simulink model "ASSIG2_vFinal"  (R2020a)
settings: Solver=FixedStepAuto  StartTime=0.0  StopTime=10.0  FixedStep=1e-3  RelTol=1e-3  EnableMultiTasking=on
undefined symbols (not defined in the file): A0, A1, D0, D1, D10, D11, D12, D13, D2, D3, D4, D5, D6, D7, D8, D9, PTA0, PTA1, PTA2, PTB2, PTB23, PTB3, PTB9, PTC16, PTC17, PTC2, PTC3, PTC4, PTD0, PTD1, PTD2, PTD3
libraries: etargetslib x22, frdmk64flib x19
settings Model: ExtModeTrigDuration=5  Creator=Nour  LastModifiedBy=Daniyal
settings OptimizationCC: EnhancedBackFolding=on  PassReuseOutputArgsAs=Individual arguments  ZeroExternalMemoryAtStartup=off  ZeroInternalMemoryAtStartup=off  MaxStackSize=64  OptimizeBlockOrder=speed  DifferentSizesBufferReuse=on  OptimizationCustomize=off  EfficientTunableParamExpr=on
settings DebuggingCC: ParameterTunabilityLossMsg=error
settings HardwareCC: ProdBitPerPointer=32  ProdBitPerSizeT=32  ProdBitPerPtrDiffT=32  ProdLargestAtomicInteger=Long  ProdLargestAtomicFloat=Double  ProdWordSize=32  ProdHWDeviceType=ARM Compatible->ARM Cortex
settings SFSimCC: MATLABDynamicMemAlloc=off
settings RTWCC: SystemTargetFile=ert.tlc  HardwareBoard=NXP FRDM-K64F  TemplateMakefile=ert_default_tmf  Toolchain=GNU Tools for ARM Embedded Processors
settings CodeAppCC: ForceParamTrailComments=on  IgnoreCustomStorageClasses=off  OperatorAnnotations=on  SimulinkDataObjDesc=on  SFDataObjDesc=on  InsertBlockDesc=on

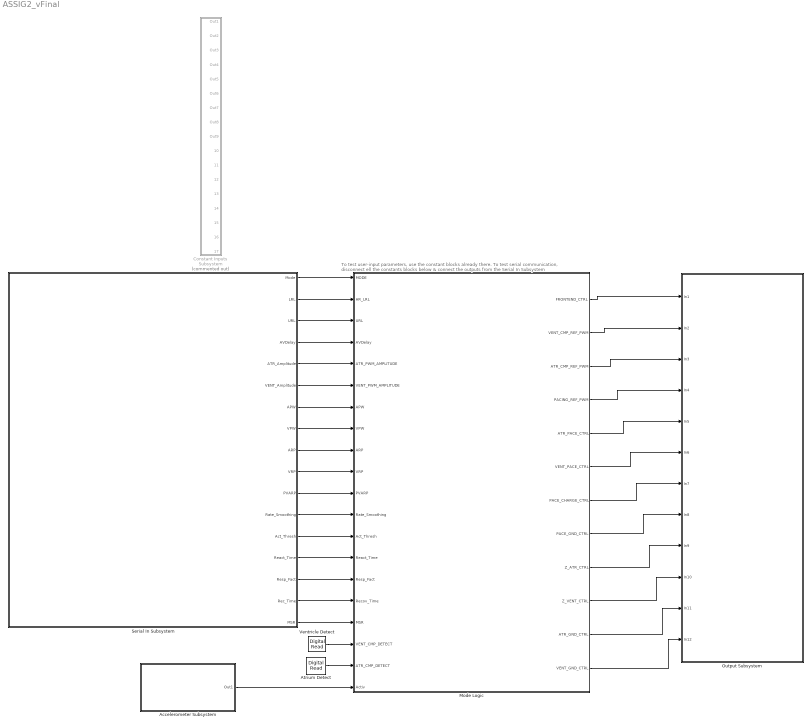
== system ASSIG2_vFinal ==
  note: To test user-input parameters, use the constant blocks already there.
      | To test serial communication, disconnect ell the constants blocks below & connect the outputs from the Serial In Subsystem
  Accelerometer Subsystem : Subsystem
  Atrium Detect : frdmk64flib/Digital Read  Whichpin=PTC16 (D0)  SampleTime=-1
  Constant Inputs Subsystem : Subsystem  Commented=on
  Mode Logic : Stateflow chart  TreatAsAtomicUnit=on
  Output Subsystem : Subsystem
  Serial In Subsystem : Subsystem
  Ventricle Detect : frdmk64flib/Digital Read  Whichpin=PTC17 (D1)  SampleTime=-1
  wires:
  Ventricle Detect/1 -> Mode Logic/18(VENT_CMP_DETECT)
  Atrium Detect/1 -> Mode Logic/19(ATR_CMP_DETECT)
  Mode Logic/1(FRONTEND_CTRL) -> Output Subsystem/1(In1)
  Mode Logic/2(VENT_CMP_REF_PWM) -> Output Subsystem/2(In2)
  Mode Logic/3(ATR_CMP_REF_PWM) -> Output Subsystem/3(In3)
  Mode Logic/4(PACING_REF_PWM) -> Output Subsystem/4(In4)
  Mode Logic/5(ATR_PACE_CTRL) -> Output Subsystem/5(In5)
  Mode Logic/6(VENT_PACE_CTRL) -> Output Subsystem/6(In6)
  Mode Logic/7(PACE_CHARGE_CTRL) -> Output Subsystem/7(In7)
  Mode Logic/8(PACE_GND_CTRL) -> Output Subsystem/8(In8)
  Mode Logic/9(Z_ATR_CTRL) -> Output Subsystem/9(In9)
  Mode Logic/10(Z_VENT_CTRL) -> Output Subsystem/10(In10)
  Mode Logic/11(ATR_GND_CTRL) -> Output Subsystem/11(In11)
  Mode Logic/12(VENT_GND_CTRL) -> Output Subsystem/12(In12)
  Serial In Subsystem/3(URL) -> Mode Logic/3(URL)
  Serial In Subsystem/4(AVDelay) -> Mode Logic/4(AVDelay)
  Serial In Subsystem/5(ATR_Amplitude) -> Mode Logic/5(ATR_PWM_AMPLITUDE)
  Serial In Subsystem/6(VENT_Amplitude) -> Mode Logic/6(VENT_PWM_AMPLITUDE)
  Serial In Subsystem/7(APW) -> Mode Logic/7(APW)
  Serial In Subsystem/8(VPW) -> Mode Logic/8(VPW)
  Serial In Subsystem/9(ARP) -> Mode Logic/9(ARP)
  Serial In Subsystem/10(VRP) -> Mode Logic/10(VRP)
  Serial In Subsystem/11(PVARP) -> Mode Logic/11(PVARP)
  Serial In Subsystem/12(Rate_Smoothing) -> Mode Logic/12(Rate_Smoothing)
  Serial In Subsystem/13(Act_Thresh) -> Mode Logic/13(Act_Thresh)
  Serial In Subsystem/14(React_Time) -> Mode Logic/14(React_Time)
  Serial In Subsystem/15(Resp_Fact) -> Mode Logic/15(Resp_Fact)
  Serial In Subsystem/16(Rec_Time) -> Mode Logic/16(Recov_Time)
  Serial In Subsystem/17(MSR) -> Mode Logic/17(MSR)
  Accelerometer Subsystem/1(Out1) -> Mode Logic/20(Activ)
  Serial In Subsystem/2(LRL) -> Mode Logic/2(HR_LRL)
  Serial In Subsystem/1(Mode) -> Mode Logic/1(MODE)

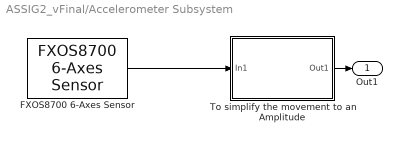
== system ASSIG2_vFinal/Accelerometer Subsystem ==
  FXOS8700 6-Axes Sensor : frdmk64flib/FXOS8700 6-Axes Sensor  Activesensor=Accelerometer only  ODR=800Hz  HybridODR=400Hz  Accelfullrange=-4g to +4g  SampleTime=-1
  To simplify the movement to an Amplitude : Subsystem
  Out1 : Outport
  wires:
  FXOS8700 6-Axes Sensor/1 -> To simplify the movement to an Amplitude/1(In1)
  To simplify the movement to an Amplitude/1(Out1) -> Out1/1

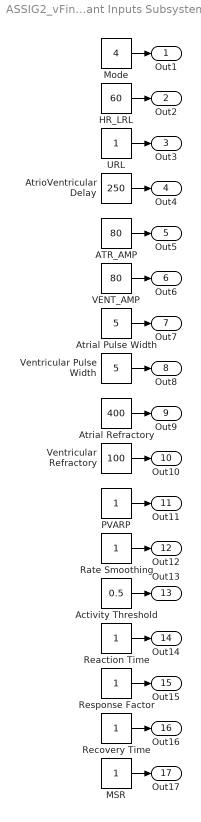
== system ASSIG2_vFinal/Constant Inputs Subsystem ==
  ATR_AMP : Constant  Value=80  OutDataTypeStr=uint8
  Activity Threshold : Constant  Value=0.5  OutDataTypeStr=single
  Atrial Pulse Width : Constant  Value=5  OutDataTypeStr=uint16
  Atrial Refractory : Constant  Value=400  OutDataTypeStr=uint16
  AtrioVentricular Delay : Constant  Value=250  OutDataTypeStr=uint16
  HR_LRL : Constant  Value=60  OutDataTypeStr=uint16
  MSR : Constant  OutDataTypeStr=uint16
  Mode : Constant  Value=4  OutDataTypeStr=uint8
  PVARP : Constant  OutDataTypeStr=uint16
  Rate Smoothing : Constant  OutDataTypeStr=uint8
  Reaction Time : Constant  OutDataTypeStr=uint16
  Recovery Time : Constant  OutDataTypeStr=uint16
  Response Factor : Constant  OutDataTypeStr=uint16
  URL : Constant  OutDataTypeStr=uint8
  VENT_AMP : Constant  Value=80  OutDataTypeStr=uint8
  Ventricular Pulse Width : Constant  Value=5  OutDataTypeStr=uint16
  Ventricular Refractory : Constant  Value=100  OutDataTypeStr=uint16
  Out1 : Outport
  Out2 : Outport  Port=2
  Out3 : Outport  Port=3
  Out4 : Outport  Port=4
  Out5 : Outport  Port=5
  Out6 : Outport  Port=6
  Out7 : Outport  Port=7
  Out8 : Outport  Port=8
  Out9 : Outport  Port=9
  Out10 : Outport  Port=10
  Out11 : Outport  Port=11
  Out12 : Outport  Port=12
  Out13 : Outport  Port=13
  Out14 : Outport  Port=14
  Out15 : Outport  Port=15
  Out16 : Outport  Port=16
  Out17 : Outport  Port=17
  wires:
  VENT_AMP/1 -> Out6/1
  Response Factor/1 -> Out15/1
  URL/1 -> Out3/1
  Recovery Time/1 -> Out16/1
  Ventricular Refractory/1 -> Out10/1
  Atrial Pulse Width/1 -> Out7/1
  Rate Smoothing/1 -> Out12/1
  Atrial Refractory/1 -> Out9/1
  Activity Threshold/1 -> Out13/1
  AtrioVentricular Delay/1 -> Out4/1
  Mode/1 -> Out1/1
  Ventricular Pulse Width/1 -> Out8/1
  Reaction Time/1 -> Out14/1
  HR_LRL/1 -> Out2/1
  PVARP/1 -> Out11/1
  MSR/1 -> Out17/1
  ATR_AMP/1 -> Out5/1

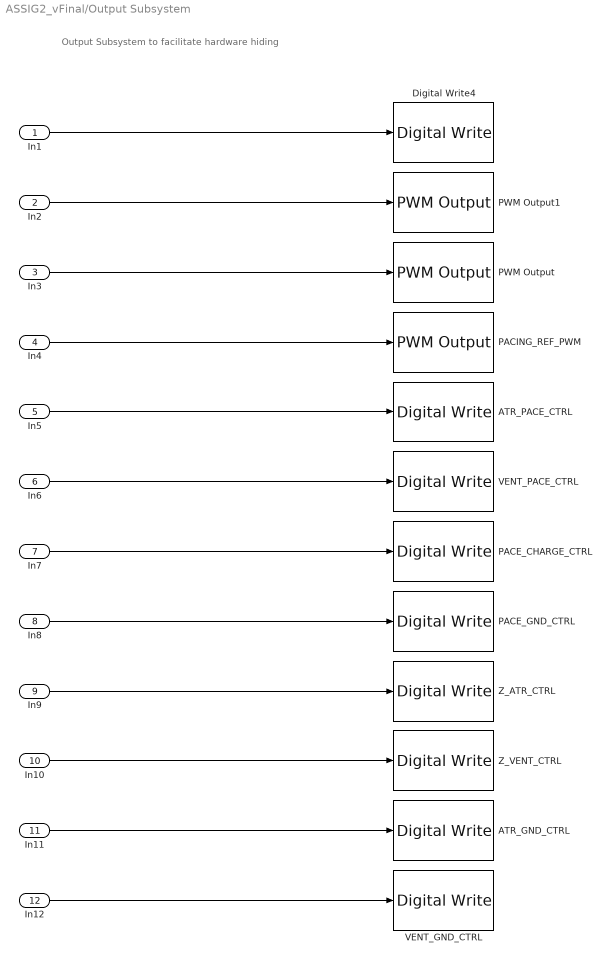
== system ASSIG2_vFinal/Output Subsystem ==
  note: Output Subsystem to facilitate hardware hiding
  In1 : Inport
  In2 : Inport  Port=2
  In3 : Inport  Port=3
  In4 : Inport  Port=4
  In5 : Inport  Port=5
  In6 : Inport  Port=6
  In7 : Inport  Port=7
  In8 : Inport  Port=8
  In9 : Inport  Port=9
  In10 : Inport  Port=10
  In11 : Inport  Port=11
  In12 : Inport  Port=12
  ATR_GND_CTRL : frdmk64flib/Digital Write  Whichpin=PTD2 (D11)
  ATR_PACE_CTRL : frdmk64flib/Digital Write  Whichpin=PTA0 (D8)
  Digital Write4 : frdmk64flib/Digital Write  Whichpin=PTD1 (D13)
  PACE_CHARGE_CTRL : frdmk64flib/Digital Write  Whichpin=PTB9 (D2)
  PACE_GND_CTRL : frdmk64flib/Digital Write  Whichpin=PTD0 (D10)
  PACING_REF_PWM : frdmk64flib/PWM Output  Whichpin=PTA2 (D5)  InitialFrequency=2000  InitialDutyCycle=80
  PWM Output : frdmk64flib/PWM Output  Whichpin=PTC2 (D6)  InitialFrequency=2000  InitialDutyCycle=20
  PWM Output1 : frdmk64flib/PWM Output  Whichpin=PTA1 (D3)  InitialFrequency=2000  InitialDutyCycle=40
  VENT_GND_CTRL : frdmk64flib/Digital Write  Whichpin=PTD3 (D12)
  VENT_PACE_CTRL : frdmk64flib/Digital Write  Whichpin=PTC4 (D9)
  Z_ATR_CTRL : frdmk64flib/Digital Write  Whichpin=PTB23 (D4)
  Z_VENT_CTRL : frdmk64flib/Digital Write  Whichpin=PTC3 (D7)
  wires:
  In7/1 -> PACE_CHARGE_CTRL/1
  In12/1 -> VENT_GND_CTRL/1
  In1/1 -> Digital Write4/1
  In4/1 -> PACING_REF_PWM/1
  In8/1 -> PACE_GND_CTRL/1
  In6/1 -> VENT_PACE_CTRL/1
  In9/1 -> Z_ATR_CTRL/1
  In10/1 -> Z_VENT_CTRL/1
  In11/1 -> ATR_GND_CTRL/1
  In2/1 -> PWM Output1/1
  In5/1 -> ATR_PACE_CTRL/1
  In3/1 -> PWM Output/1

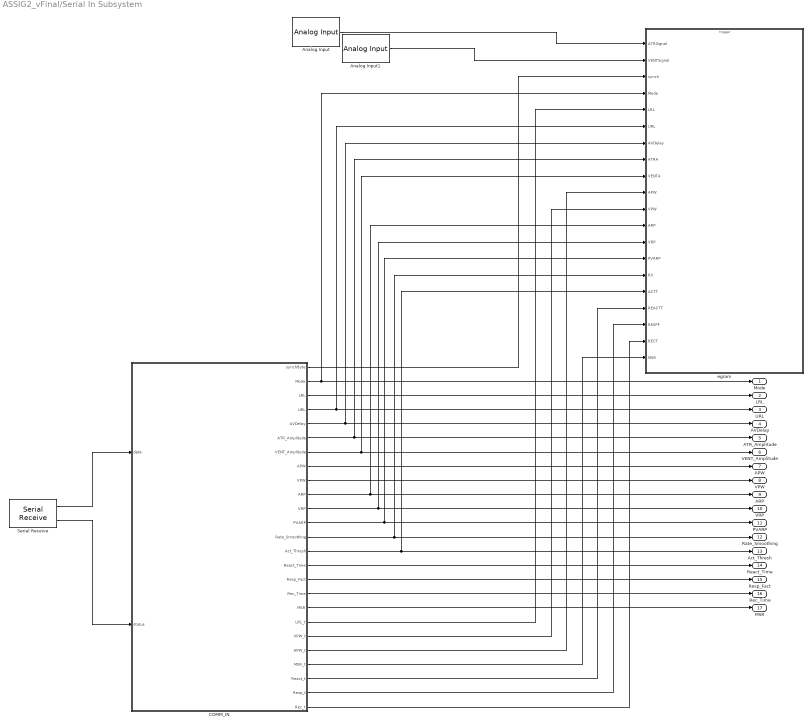
== system ASSIG2_vFinal/Serial In Subsystem ==
  Analog Input : frdmk64flib/Analog Input  Whichpin=PTB2 (A0)  SampleTime=-1
  Analog Input1 : frdmk64flib/Analog Input  Whichpin=PTB3 (A1)  SampleTime=-1
  COMM_IN : Stateflow chart  TreatAsAtomicUnit=on
  Serial Receive : frdmk64flib/Serial Receive  SCIModule=0  Baudrate=uint32(9600)  Parity=None  StopBits=1  HardwareFlowControl=None  ByteOrder=LittleEndian  DataType=uint8  DataLength=26  BlockingMode=off  OutputStatus=on  SampleTime=-1
  egram : Subsystem
  Mode : Outport
  LRL : Outport  Port=2
  URL : Outport  Port=3
  AVDelay : Outport  Port=4
  ATR_Amplitude : Outport  Port=5
  VENT_Amplitude : Outport  Port=6
  APW : Outport  Port=7
  VPW : Outport  Port=8
  ARP : Outport  Port=9
  VRP : Outport  Port=10
  PVARP : Outport  Port=11
  Rate_Smoothing : Outport  Port=12
  Act_Thresh : Outport  Port=13
  React_Time : Outport  Port=14
  Resp_Fact : Outport  Port=15
  Rec_Time : Outport  Port=16
  MSR : Outport  Port=17
  wires:
  Serial Receive/1 -> COMM_IN/1(data)
  Serial Receive/2 -> COMM_IN/2(status)
  Analog Input/1 -> egram/1(ATRSignal)
  Analog Input1/1 -> egram/2(VENTSignal)
  COMM_IN/2(Mode) -> Mode/1, egram/4(Mode)
  COMM_IN/3(LRL) -> LRL/1
  COMM_IN/4(URL) -> URL/1, egram/6(URL)
  COMM_IN/5(AVDelay) -> AVDelay/1, egram/7(AVDelay)
  COMM_IN/6(ATR_Amplitude) -> egram/8(ATRA), ATR_Amplitude/1
  COMM_IN/7(VENT_Amplitude) -> egram/9(VENTA), VENT_Amplitude/1
  COMM_IN/8(APW) -> APW/1
  COMM_IN/9(VPW) -> VPW/1
  COMM_IN/10(ARP) -> egram/12(ARP), ARP/1
  COMM_IN/18(MSR) -> MSR/1
  COMM_IN/17(Rec_Time) -> Rec_Time/1
  COMM_IN/16(Resp_Fact) -> Resp_Fact/1
  COMM_IN/15(React_Time) -> React_Time/1
  COMM_IN/14(Act_Thresh) -> egram/16(ACTT), Act_Thresh/1
  COMM_IN/13(Rate_Smoothing) -> egram/15(RS), Rate_Smoothing/1
  COMM_IN/12(PVARP) -> egram/14(PVARP), PVARP/1
  COMM_IN/11(VRP) -> egram/13(VRP), VRP/1
  COMM_IN/1(synchByte) -> egram/3(synch)
  COMM_IN/19(LRL_t) -> egram/5(LRL)
  COMM_IN/20(VPW_t) -> egram/11(VPW)
  COMM_IN/21(APW_t) -> egram/10(APW)
  COMM_IN/23(React_t) -> egram/17(REACTT)
  COMM_IN/24(Resp_t) -> egram/18(RESPF)
  COMM_IN/25(Rec_t) -> egram/19(RECT)
  COMM_IN/22(MSR_t) -> egram/20(MSR)

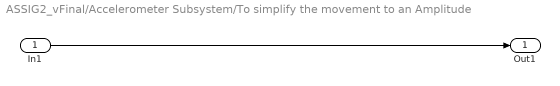
== system ASSIG2_vFinal/Accelerometer Subsystem/To simplify the movement to an Amplitude ==
  In1 : Inport
  Out1 : Outport
  wires:
  In1/1 -> Out1/1

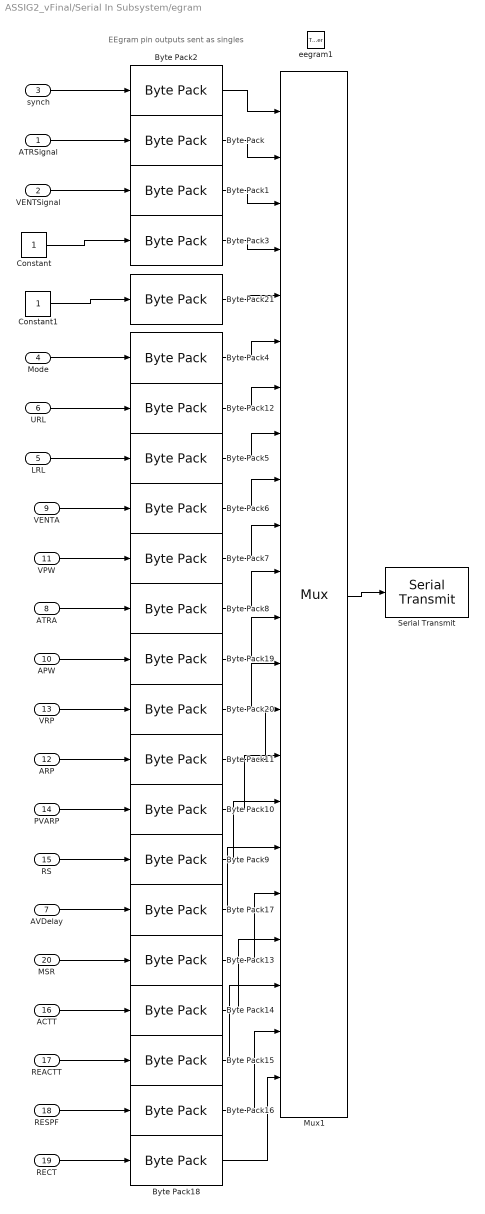
== system ASSIG2_vFinal/Serial In Subsystem/egram ==
  note: EEgram pin outputs sent as singles
  ATRSignal : Inport
  VENTSignal : Inport  Port=2
  synch : Inport  Port=3
  Mode : Inport  Port=4
  LRL : Inport  Port=5
  URL : Inport  Port=6
  AVDelay : Inport  Port=7
  ATRA : Inport  Port=8
  VENTA : Inport  Port=9
  APW : Inport  Port=10
  VPW : Inport  Port=11
  ARP : Inport  Port=12
  VRP : Inport  Port=13
  PVARP : Inport  Port=14
  RS : Inport  Port=15
  ACTT : Inport  Port=16
  REACTT : Inport  Port=17
  RESPF : Inport  Port=18
  RECT : Inport  Port=19
  MSR : Inport  Port=20
  eegram1 : TriggerPort  TriggerType=function-call  IsSimulinkFunction=on  FunctionName=eegram1  VariantControl=Variant  PortDimensions=1
  Byte Pack : etargetslib/Byte Pack  datatypes={'double'}  byteAlign=1
  Byte Pack1 : etargetslib/Byte Pack  datatypes={'double'}  byteAlign=1
  Byte Pack{3,10..11,17,20} (5 alike) : etargetslib/Byte Pack  datatypes={'uint16'}  byteAlign=1
  Byte Pack{2,4..9,12..13,15..16,18..19} (13 alike) : etargetslib/Byte Pack  datatypes={'uint8'}  byteAlign=1
  Byte Pack14 : etargetslib/Byte Pack  datatypes={'single'}  byteAlign=1
  Byte Pack21 : etargetslib/Byte Pack  datatypes={'single'}  byteAlign=1
  Constant : Constant  OutDataTypeStr=uint16
  Constant1 : Constant  OutDataTypeStr=single
  Mux1 : Mux  Inputs=22
  Serial Transmit : frdmk64flib/Serial Transmit  SCIModule=0  Baudrate=uint32(9600)  Parity=None  StopBits=1  HardwareFlowControl=None  ByteOrder=LittleEndian  BlockingMode=on  OutputStatus=off
  wires:
  ATRSignal/1 -> Byte Pack/1
  VENTSignal/1 -> Byte Pack1/1
  Mode/1 -> Byte Pack4/1
  ARP/1 -> Byte Pack11/1
  synch/1 -> Byte Pack2/1
  ACTT/1 -> Byte Pack14/1
  PVARP/1 -> Byte Pack10/1
  VENTA/1 -> Byte Pack6/1
  MSR/1 -> Byte Pack13/1
  AVDelay/1 -> Byte Pack17/1
  REACTT/1 -> Byte Pack15/1
  LRL/1 -> Byte Pack5/1
  VRP/1 -> Byte Pack20/1
  ATRA/1 -> Byte Pack8/1
  APW/1 -> Byte Pack19/1
  RS/1 -> Byte Pack9/1
  VPW/1 -> Byte Pack7/1
  URL/1 -> Byte Pack12/1
  RESPF/1 -> Byte Pack16/1
  RECT/1 -> Byte Pack18/1
  Byte Pack2/1 -> Mux1/1
  Byte Pack/1 -> Mux1/2
  Byte Pack1/1 -> Mux1/3
  Mux1/1 -> Serial Transmit/1
  Constant/1 -> Byte Pack3/1
  Byte Pack3/1 -> Mux1/4
  Byte Pack21/1 -> Mux1/5
  Byte Pack4/1 -> Mux1/6
  Byte Pack12/1 -> Mux1/7
  Byte Pack5/1 -> Mux1/8
  Byte Pack6/1 -> Mux1/9
  Byte Pack7/1 -> Mux1/10
  Byte Pack8/1 -> Mux1/11
  Byte Pack19/1 -> Mux1/12
  Byte Pack20/1 -> Mux1/13
  Byte Pack11/1 -> Mux1/14
  Byte Pack10/1 -> Mux1/15
  Byte Pack9/1 -> Mux1/16
  Byte Pack17/1 -> Mux1/17
  Byte Pack13/1 -> Mux1/18
  Byte Pack14/1 -> Mux1/19
  Byte Pack15/1 -> Mux1/20
  Byte Pack16/1 -> Mux1/21
  Byte Pack18/1 -> Mux1/22
  Constant1/1 -> Byte Pack21/1

== stateflow chart ASSIG2_vFinal/Serial In Subsystem/COMM_IN ==
  state SET_PARAM
    entry:
    %% initial typecast of values through
    %% serial communication
    Mode = typecast(data(3), 'uint8');
    URL = typecast(data(4), 'uint8');
    LRL_t = typecast(data(5), 'uint8');
    VENT_Amplitude = typecast(data(6), 'uint8');
    VPW_t = typecast(data(7), 'uint8');
    ATR_Amplitude = typecast(data(8), 'uint8');
    APW_t = typecast(data(9), 'uint8');
    VRP = typecast(data(10:11), 'uint16');
    ARP = typecast(data(12:13), 'uint16');
    PVARP = typecast(data(14:15), 'uint16');
    Rate_Smoothing = typecast(data(16), 'uint8');
    AVDelay = typecast(data(17: 18), 'uint16');
    MSR_t = typecast(data(19), 'uint8');
    Act_Thresh = typecast(data(20:23), 'single');
    React_t = typecast(data(24), 'uint8');
    Resp_t = typecast(data(25), 'uint8');
    Rec_t = typecast(data(26), 'uint8');
  state RETYPECAST
    entry:
    %% 2ndary typecast
    LRL  = 2*uint16(LRL_t);
    VPW  = 2*uint16(VPW_t);
    APW  = 2*uint16(APW_t);
    MSR  = 2*uint16(MSR_t);
    React_Time = 2*uint16(React_t);
    Resp_Fact = 2*uint16(Resp_t);
    Rec_Time = 2*uint16(Rec_t);
  state INITIAL
    %% Setting initial, default values of parameters
    entry:
    Mode = 0;
    URL = 0;
    LRL = 0;
    VENT_Amplitude = 0;
    VPW = 0;
    ATR_Amplitude = 0;
    APW = 0;
    VRP = 0;
    ARP = 0;
    PVARP = 0;
    Rate_Smoothing = 0;
    AVDelay = 0;
    MSR = 0;
    Act_Thresh = 0;
    React_Time = 0;
    Resp_Fact = 0;
    Rec_Time = 0;
  state STANDBY
    entry:
    %% Waiting for COM
    %% function code values;
    %% 55 -> set params
    %% 22 -> eegram
    %% 33 -> return params
    synchByte = typecast(data(1), 'uint8');
    %% fn_code = typecast(data(2), 'uint8');
  state EEGRAM
    entry:
    eegram1();
  (junction 15) -> SET_PARAM [order 2] : [data(2) == hex2dec('55')]
  SET_PARAM -> RETYPECAST
  RETYPECAST -> STANDBY
  (default) -> INITIAL
  (junction 13) -> STANDBY [order 2]
  INITIAL -> STANDBY
  STANDBY -> (junction 13) : [status == 0]
  (junction 13) -> (junction 15) [order 1] : [data(1) == hex2dec('16')]
  (junction 15) -> EEGRAM [order 1] : [data(2) == hex2dec('22')]
  EEGRAM -> STANDBY
  data: synchByte output uint8; data input uint8 size=[26;1]; status input uint8 size=[1;1]; Mode output uint8; LRL output uint16; URL output uint8; AVDelay output uint16; ATR_Amplitude output uint8; VENT_Amplitude output uint8; APW output uint16; VPW output uint16; ARP output uint16; VRP output uint16; PVARP output uint16; Rate_Smoothing output uint8; Act_Thresh output single; React_Time output uint16; Resp_Fact output uint16; Rec_Time output uint16; MSR output uint16; LRL_t output uint8; VPW_t output uint8; APW_t output uint8; MSR_t output uint8; React_t output uint8; Resp_t output uint8; Rec_t output uint8

== stateflow chart ASSIG2_vFinal/Mode Logic ==
  state AOO
    state ChargeATR
      entry:
      ATR_PACE_CTRL = false;
      VENT_PACE_CTRL = false;
      PACING_REF_PWM = ATR_PWM_AMPLITUDE;
      PACE_CHARGE_CTRL = true;
      %Discharging Blocking Capacitor
      PACE_GND_CTRL = true;
      VENT_PACE_CTRL = false;
      Z_ATR_CTRL = false;
      Z_VENT_CTRL = false;
      %% ATR_PACE_CTRL = false;
      ATR_GND_CTRL = true;
      VENT_GND_CTRL = false;
    state PaceATR
      entry:
      PACE_CHARGE_CTRL = false;
      PACE_GND_CTRL = true;
      ATR_PACE_CTRL = true;
      ATR_GND_CTRL = false;
      Z_ATR_CTRL = false;
      Z_VENT_CTRL = false;
      VENT_GND_CTRL = false;
      VENT_PACE_CTRL = false;
    (default) -> ChargeATR
    ChargeATR -> PaceATR : [after((60000 / HR_LRL - APW), msec)]
    PaceATR -> ChargeATR : [after(APW, msec)]
  state VOO
    state ChargeVENT
      %% Charge C22, Discharge C21
      entry:
      ATR_PACE_CTRL = false;
      VENT_PACE_CTRL = false;
      PACING_REF_PWM = VENT_PWM_AMPLITUDE;
      PACE_CHARGE_CTRL = true;
      %Dishcharging Blocking Capacitor
      PACE_GND_CTRL = true;
      Z_ATR_CTRL = false;
      Z_VENT_CTRL = false;
      ATR_GND_CTRL = false;
      VENT_GND_CTRL = true;
    state PaceVENT
      entry:
      PACE_CHARGE_CTRL = false;
      PACE_GND_CTRL = true;
      ATR_PACE_CTRL = false;
      ATR_GND_CTRL = false;
      Z_ATR_CTRL = false;
      Z_VENT_CTRL = false;
      VENT_GND_CTRL = false;
      VENT_PACE_CTRL = true;
    (default) -> ChargeVENT
    ChargeVENT -> PaceVENT : [after((60000 / HR_LRL - VPW), msec)]
    PaceVENT -> ChargeVENT : [after(VPW, msec)]
  state Entry
    %% MODE Values:
    %% verify means it hasn't been checked
    %% 1: AOO
    %% 2: VOO
    %% 3: AAI
    %% 4: VVI
    %% 5: DOO
    %% 6: AOOR verify
    %% 7: VOOR verify
    %% 8: AAIR verify
    %% 9:  VVIR verify
    %% 10: DOOR verify
    entry:
    ATR_CMP_REF_PWM = 60;
    VENT_CMP_REF_PWM = 60;
    delay = 0;
  state AAI
    state Charge
      entry:
      ATR_PACE_CTRL = false;
      VENT_PACE_CTRL = false;
      PACING_REF_PWM = ATR_PWM_AMPLITUDE;
      PACE_CHARGE_CTRL = true;
      %Discharging Blocking Capacitor
      PACE_GND_CTRL = true;
      VENT_PACE_CTRL = false;
      Z_ATR_CTRL = false;
      Z_VENT_CTRL = false;
      %% ATR_PACE_CTRL = false;
      ATR_GND_CTRL = true;
      VENT_GND_CTRL = false;
      FRONTEND_CTRL = true;
    state Pace
      entry:
      PACE_CHARGE_CTRL = false;
      PACE_GND_CTRL = true;
      ATR_PACE_CTRL = true;
      ATR_GND_CTRL = false;
      Z_ATR_CTRL = false;
      Z_VENT_CTRL = false;
      VENT_GND_CTRL = false;
      VENT_PACE_CTRL = false;
      %% FRONTEND_CTRL = true;
    state Refractor
      entry:
      ATR_PACE_CTRL = false;
      VENT_PACE_CTRL = false;
      PACING_REF_PWM = ATR_PWM_AMPLITUDE;
      PACE_CHARGE_CTRL = true;
      %Discharging Blocking Capacitor
      PACE_GND_CTRL = true;
      VENT_PACE_CTRL = false;
      Z_ATR_CTRL = false;
      Z_VENT_CTRL = false;
      %% ATR_PACE_CTRL = false;
      ATR_GND_CTRL = true;
      VENT_GND_CTRL = false;
      %% FRONTEND_CTRL = true;
    (default) -> AAI.Charge
    AAI.Charge -> AAI.Pace [order 1] : [after((60000 / HR_LRL - ARP - delay), msec)]
    AAI.Charge -> AAI.Refractor [order 2] : [ATR_CMP_DETECT == true]{delay = 0}
    AAI.Refractor -> AAI.Charge : [after(ARP, msec)]
    AAI.Pace -> AAI.Refractor : [after(APW, msec)]{delay = APW}
  state DOOR
    state ATRCharge
      state CHARGE
        entry:
        ATR_PACE_CTRL = false;
        VENT_PACE_CTRL = false;
        PACING_REF_PWM = ATR_PWM_AMPLITUDE;
        PACE_CHARGE_CTRL = true;
        %Discharging Blocking Capacitor
        PACE_GND_CTRL = true;
        VENT_PACE_CTRL = false;
        Z_ATR_CTRL = false;
        Z_VENT_CTRL = false;
        %% ATR_PACE_CTRL = false;
        ATR_GND_CTRL = true;
        VENT_GND_CTRL = false;
        Activ_Rate = single(sqrt(abs(Activ(1))^2+abs(Activ(2))^2+abs(Activ(3))^2));
      state ENTRY_STATE1
        prev_HR_LRL = HR_LRLR;
        %% equation to get Reqi_HR_LRL
        ReqI_HR_LRL = ceil((MSR - HR_LRL) * (Resp_Fact / 16) + HR_LRL);
        %% Final_dHR is just HR_LRL
        ReqD_HR_LRL = HR_LRL;
      state Increment_HR1
        %% deltaI_HR = uint16(Activ_Rate * 10);
        deltaI_HR = ceil((ReqI_HR_LRL - prev_HR_LRL) + (uint16(round(Activ_Rate)) ));
        HR_LRLR = ceil(prev_HR_LRL + (deltaI_HR * 10 / React_Time));
      state Decrement_HR1
        deltaD_HR = floor((MSR + prev_HR_LRL)) / 2 - ReqD_HR_LRL;
        HR_LRLR = floor(prev_HR_LRL - (deltaD_HR * 10) / ( Recov_Time*60))
      state Maintain_HR1
        HR_LRLR = prev_HR_LRL;
      (default) -> DOOR.ATRCharge.CHARGE
      DOOR.ATRCharge.CHARGE -> DOOR.ATRCharge.ENTRY_STATE1
      DOOR.ATRCharge.ENTRY_STATE1 -> (junction 401) [order 1] : [Activ_Rate >= Act_Thresh]
      DOOR.ATRCharge.ENTRY_STATE1 -> (junction 402) [order 2] : [Activ_Rate< Act_Thresh]
      (junction 401) -> DOOR.ATRCharge.Maintain_HR1 [order 2] : [prev_HR_LRL >= ReqI_HR_LRL]
      (junction 401) -> DOOR.ATRCharge.Increment_HR1 [order 1] : [prev_HR_LRL < ReqI_HR_LRL]
      (junction 402) -> DOOR.ATRCharge.Maintain_HR1 [order 1] : [prev_HR_LRL <= ReqD_HR_LRL]
      (junction 402) -> DOOR.ATRCharge.Decrement_HR1 [order 2] : [prev_HR_LRL > ReqD_HR_LRL]
    state ATRPace
      entry:
      entry:
      PACE_CHARGE_CTRL = false;
      PACE_GND_CTRL = true;
      ATR_PACE_CTRL = true;
      ATR_GND_CTRL = false;
      Z_ATR_CTRL = false;
      Z_VENT_CTRL = false;
      VENT_GND_CTRL = false;
      VENT_PACE_CTRL = false;
    state VENTCharge
      %% Charge C22, Discharge C21
      entry:
      ATR_PACE_CTRL = false;
      VENT_PACE_CTRL = false;
      PACING_REF_PWM = VENT_PWM_AMPLITUDE;
      PACE_CHARGE_CTRL = true;
      %Dishcharging Blocking Capacitor
      PACE_GND_CTRL = true;
      Z_ATR_CTRL = false;
      Z_VENT_CTRL = false;
      ATR_GND_CTRL = false;
      VENT_GND_CTRL = true;
    state VentPace
      entry:
      PACE_CHARGE_CTRL = false;
      PACE_GND_CTRL = true;
      ATR_PACE_CTRL = false;
      ATR_GND_CTRL = false;
      Z_ATR_CTRL = false;
      Z_VENT_CTRL = false;
      VENT_GND_CTRL = false;
      VENT_PACE_CTRL = true;
    (default) -> DOOR.ATRCharge : {HR_LRLR = HR_LRL}
    DOOR.ATRCharge -> DOOR.ATRPace : [after((60000 / HR_LRLR - AVDelay - APW - VPW), msec)]
    DOOR.ATRPace -> DOOR.VENTCharge : [after(APW, msec)]
    DOOR.VentPace -> DOOR.ATRCharge : [after(VPW, msec)]
    DOOR.VENTCharge -> DOOR.VentPace : [after(AVDelay, msec)]
  state VVI
    state Charge
      %% Charge C22, Discharge C21
      entry:
      ATR_PACE_CTRL = false;
      VENT_PACE_CTRL = false;
      PACING_REF_PWM = VENT_PWM_AMPLITUDE;
      PACE_CHARGE_CTRL = true;
      %Dishcharging Blocking Capacitor
      PACE_GND_CTRL = true;
      VENT_PACE_CTRL = false;
      Z_ATR_CTRL = false;
      Z_VENT_CTRL = false;
      ATR_GND_CTRL = false;
      VENT_GND_CTRL = true;
      FRONTEND_CTRL = true;
    state Pace
      entry:
      PACE_CHARGE_CTRL = false;
      PACE_GND_CTRL = true;
      ATR_PACE_CTRL = false;
      ATR_GND_CTRL = false;
      Z_ATR_CTRL = false;
      Z_VENT_CTRL = false;
      VENT_GND_CTRL = false;
      VENT_PACE_CTRL = true;
      %FRONTEND_CTRL = true;
    state Refractor
      %% Charge C22, Discharge C21
      entry:
      ATR_PACE_CTRL = false;
      VENT_PACE_CTRL = false;
      PACING_REF_PWM = VENT_PWM_AMPLITUDE;
      PACE_CHARGE_CTRL = true;
      %Dishcharging Blocking Capacitor
      PACE_GND_CTRL = true;
      VENT_PACE_CTRL = false;
      Z_ATR_CTRL = false;
      Z_VENT_CTRL = false;
      ATR_GND_CTRL = false;
      VENT_GND_CTRL = true;
      %FRONTEND_CTRL = true;
    (default) -> VVI.Charge
    VVI.Charge -> VVI.Pace [order 1] : [after((60000 / HR_LRL - VRP - delay), msec)]
    VVI.Charge -> VVI.Refractor [order 2] : [VENT_CMP_DETECT == true]{delay = 0}
    VVI.Refractor -> VVI.Charge : [after(VRP+VPW, msec)]
    VVI.Pace -> VVI.Refractor : [after(VPW, msec)]{delay = VPW}
  state VVIR
    state Charge
      state CHARGE
        %% Charge C22, Discharge C21
        entry:
        ATR_PACE_CTRL = false;
        VENT_PACE_CTRL = false;
        PACING_REF_PWM = VENT_PWM_AMPLITUDE;
        PACE_CHARGE_CTRL = true;
        %Dishcharging Blocking Capacitor
        PACE_GND_CTRL = true;
        Z_ATR_CTRL = false;
        Z_VENT_CTRL = false;
        ATR_GND_CTRL = false;
        VENT_GND_CTRL = true;
        FRONTEND_CTRL = true;
        Activ_Rate = single(sqrt(abs(Activ(1))^2+abs(Activ(2))^2+abs(Activ(3))^2));
      state ENTRY_STATE1
        prev_HR_LRL = HR_LRLR;
        %% equation to get Reqi_HR_LRL
        ReqI_HR_LRL = ceil((MSR - HR_LRL) * (Resp_Fact / 16) + HR_LRL);
        %% Final_dHR is just HR_LRL
        ReqD_HR_LRL = HR_LRL;
      state Increment_HR1
        %% deltaI_HR = uint16(Activ_Rate * 10);
        deltaI_HR = ceil((ReqI_HR_LRL - prev_HR_LRL) + (uint16(round(Activ_Rate)) ));
        HR_LRLR = ceil(prev_HR_LRL + (deltaI_HR * 10 / React_Time));
      state Decrement_HR1
        deltaD_HR = floor((MSR + prev_HR_LRL)) / 2 - ReqD_HR_LRL;
        HR_LRLR = floor(prev_HR_LRL - (deltaD_HR * 10) / ( Recov_Time*60))
      state Maintain_HR1
        HR_LRLR = prev_HR_LRL;
      (default) -> VVIR.Charge.CHARGE
      VVIR.Charge.CHARGE -> VVIR.Charge.ENTRY_STATE1
      VVIR.Charge.ENTRY_STATE1 -> (junction 385) [order 1] : [Activ_Rate >= Act_Thresh]
      VVIR.Charge.ENTRY_STATE1 -> (junction 386) [order 2] : [Activ_Rate< Act_Thresh]
      (junction 385) -> VVIR.Charge.Maintain_HR1 [order 2] : [prev_HR_LRL >= ReqI_HR_LRL]
      (junction 385) -> VVIR.Charge.Increment_HR1 [order 1] : [prev_HR_LRL < ReqI_HR_LRL]
      (junction 386) -> VVIR.Charge.Maintain_HR1 [order 1] : [prev_HR_LRL <= ReqD_HR_LRL]
      (junction 386) -> VVIR.Charge.Decrement_HR1 [order 2] : [prev_HR_LRL > ReqD_HR_LRL]
    state Pace
      entry:
      PACE_CHARGE_CTRL = false;
      PACE_GND_CTRL = true;
      ATR_PACE_CTRL = false;
      ATR_GND_CTRL = false;
      Z_ATR_CTRL = false;
      Z_VENT_CTRL = false;
      VENT_GND_CTRL = false;
      VENT_PACE_CTRL = true;
      %% FRONTEND_CTRL = true;
    state Refractor
      %% Charge C22, Discharge C21
      entry:
      ATR_PACE_CTRL = false;
      VENT_PACE_CTRL = false;
      PACING_REF_PWM = VENT_PWM_AMPLITUDE;
      PACE_CHARGE_CTRL = true;
      %Dishcharging Blocking Capacitor
      PACE_GND_CTRL = true;
      Z_ATR_CTRL = false;
      Z_VENT_CTRL = false;
      ATR_GND_CTRL = false;
      VENT_GND_CTRL = true;
      %% FRONTEND_CTRL = true;
    (default) -> VVIR.Charge : {HR_LRLR = HR_LRL}
    VVIR.Charge -> VVIR.Refractor [order 2] : [VENT_CMP_DETECT == true]{delay = 0}
    VVIR.Charge -> VVIR.Pace [order 1] : [after((60000 / HR_LRLR - VRP - delay), msec)]
    VVIR.Refractor -> VVIR.Charge : [after(VRP, msec)]
    VVIR.Pace -> VVIR.Refractor : [after(VPW, msec)]{delay = VPW}
  state AAIR
    state Charge_AAIR
      state CHARGE
        entry:
        ATR_PACE_CTRL = false;
        VENT_PACE_CTRL = false;
        PACING_REF_PWM = ATR_PWM_AMPLITUDE;
        PACE_CHARGE_CTRL = true;
        %Discharging Blocking Capacitor
        PACE_GND_CTRL = true;
        VENT_PACE_CTRL = false;
        Z_ATR_CTRL = false;
        Z_VENT_CTRL = false;
        %% ATR_PACE_CTRL = false;
        ATR_GND_CTRL = true;
        VENT_GND_CTRL = false;
        FRONTEND_CTRL = true;
        Activ_Rate = single(sqrt(abs(Activ(1))^2+abs(Activ(2))^2+abs(Activ(3))^2));
      state ENTRY_STATE1
        prev_HR_LRL = HR_LRLR;
        %% equation to get Reqi_HR_LRL
        ReqI_HR_LRL = ceil((MSR - HR_LRL) * (Resp_Fact / 16) + HR_LRL);
        %% Final_dHR is just HR_LRL
        ReqD_HR_LRL = HR_LRL;
      state Increment_HR1
        %% deltaI_HR = uint16(Activ_Rate * 10);
        deltaI_HR = ceil((ReqI_HR_LRL - prev_HR_LRL) + (uint16(round(Activ_Rate)) ));
        HR_LRLR = ceil(prev_HR_LRL + (deltaI_HR * 10 / React_Time));
      state Decrement_HR1
        deltaD_HR = floor((MSR + prev_HR_LRL)) / 2 - ReqD_HR_LRL;
        HR_LRLR = floor(prev_HR_LRL - (deltaD_HR * 10) / ( Recov_Time*60))
      state Maintain_HR1
        HR_LRLR = prev_HR_LRL;
      (default) -> AAIR.Charge_AAIR.CHARGE
      AAIR.Charge_AAIR.CHARGE -> AAIR.Charge_AAIR.ENTRY_STATE1
      AAIR.Charge_AAIR.ENTRY_STATE1 -> (junction 363) [order 1] : [Activ_Rate >= Act_Thresh]
      AAIR.Charge_AAIR.ENTRY_STATE1 -> (junction 362) [order 2] : [Activ_Rate< Act_Thresh]
      (junction 363) -> AAIR.Charge_AAIR.Maintain_HR1 [order 2] : [prev_HR_LRL >= ReqI_HR_LRL]
      (junction 363) -> AAIR.Charge_AAIR.Increment_HR1 [order 1] : [prev_HR_LRL < ReqI_HR_LRL]
      (junction 362) -> AAIR.Charge_AAIR.Maintain_HR1 [order 1] : [prev_HR_LRL <= ReqD_HR_LRL]
      (junction 362) -> AAIR.Charge_AAIR.Decrement_HR1 [order 2] : [prev_HR_LRL > ReqD_HR_LRL]
    state Pace
      entry:
      PACE_CHARGE_CTRL = false;
      PACE_GND_CTRL = true;
      ATR_PACE_CTRL = true;
      ATR_GND_CTRL = false;
      Z_ATR_CTRL = false;
      Z_VENT_CTRL = false;
      VENT_GND_CTRL = false;
      VENT_PACE_CTRL = false;
      %% FRONTEND_CTRL = true;
    state Refractor
      entry:
      ATR_PACE_CTRL = false;
      VENT_PACE_CTRL = false;
      PACING_REF_PWM = ATR_PWM_AMPLITUDE;
      PACE_CHARGE_CTRL = true;
      %Discharging Blocking Capacitor
      PACE_GND_CTRL = true;
      VENT_PACE_CTRL = false;
      Z_ATR_CTRL = false;
      Z_VENT_CTRL = false;
      %% ATR_PACE_CTRL = false;
      ATR_GND_CTRL = true;
      VENT_GND_CTRL = false;
      %% FRONTEND_CTRL = true;
    (default) -> Charge_AAIR : {HR_LRLR = HR_LRL}
    Charge_AAIR -> AAIR.Pace [order 1] : [after((60000 / HR_LRLR - ARP - delay), msec)]
    Charge_AAIR -> AAIR.Refractor [order 2] : [ATR_CMP_DETECT == true]{delay = 0}
    AAIR.Refractor -> Charge_AAIR : [after(ARP, msec)]
    AAIR.Pace -> AAIR.Refractor : [after(APW, msec)]{delay = APW}
  state DOO
    state ATRCharge
      entry:
      ATR_PACE_CTRL = false;
      VENT_PACE_CTRL = false;
      PACING_REF_PWM = ATR_PWM_AMPLITUDE;
      PACE_CHARGE_CTRL = true;
      %Discharging Blocking Capacitor
      PACE_GND_CTRL = true;
      VENT_PACE_CTRL = false;
      Z_ATR_CTRL = false;
      Z_VENT_CTRL = false;
      %% ATR_PACE_CTRL = false;
      ATR_GND_CTRL = true;
      VENT_GND_CTRL = false;
    state ATRPace
      entry:
      entry:
      PACE_CHARGE_CTRL = false;
      PACE_GND_CTRL = true;
      ATR_PACE_CTRL = true;
      ATR_GND_CTRL = false;
      Z_ATR_CTRL = false;
      Z_VENT_CTRL = false;
      VENT_GND_CTRL = false;
      VENT_PACE_CTRL = false;
    state VENTCharge
      %% Charge C22, Discharge C21
      entry:
      ATR_PACE_CTRL = false;
      VENT_PACE_CTRL = false;
      PACING_REF_PWM = VENT_PWM_AMPLITUDE;
      PACE_CHARGE_CTRL = true;
      %Dishcharging Blocking Capacitor
      PACE_GND_CTRL = true;
      Z_ATR_CTRL = false;
      Z_VENT_CTRL = false;
      ATR_GND_CTRL = false;
      VENT_GND_CTRL = true;
    state VentPace
      entry:
      PACE_CHARGE_CTRL = false;
      PACE_GND_CTRL = true;
      ATR_PACE_CTRL = false;
      ATR_GND_CTRL = false;
      Z_ATR_CTRL = false;
      Z_VENT_CTRL = false;
      VENT_GND_CTRL = false;
      VENT_PACE_CTRL = true;
    (default) -> DOO.ATRCharge
    DOO.ATRCharge -> DOO.ATRPace : [after((60000 / HR_LRL - AVDelay - APW - VPW), msec)]
    DOO.ATRPace -> DOO.VENTCharge : [after(APW, msec)]
    DOO.VentPace -> DOO.ATRCharge : [after(VPW, msec)]
    DOO.VENTCharge -> DOO.VentPace : [after(AVDelay, msec)]
  state VOOR
    state VOOR_CHARGE
      state Charge
        %% Charge C22, Discharge C21
        entry:
        ATR_PACE_CTRL = false;
        VENT_PACE_CTRL = false;
        PACING_REF_PWM = VENT_PWM_AMPLITUDE;
        PACE_CHARGE_CTRL = true;
        %Dishcharging Blocking Capacitor
        PACE_GND_CTRL = true;
        VENT_PACE_CTRL = false;
        Z_ATR_CTRL = false;
        Z_VENT_CTRL = false;
        ATR_GND_CTRL = false;
        VENT_GND_CTRL = true;
        Activ_Rate = single(sqrt(abs(Activ(1))^2+abs(Activ(2))^2+abs(Activ(3))^2));
      state ENTRY_STATE2
        prev_HR_LRL = HR_LRLR;
        %% equation to get Reqi_HR_LRL
        ReqI_HR_LRL = ceil((MSR - HR_LRL) * (Resp_Fact / 16) + HR_LRL);
        %% Final_dHR is just HR_LRL
        ReqD_HR_LRL = HR_LRL;
      state Increment_HR2
        %% deltaI_HR = uint16(Activ_Rate * 10);
        deltaI_HR = ceil((ReqI_HR_LRL - prev_HR_LRL) + (uint16(round(Activ_Rate)) ));
        HR_LRLR = ceil(prev_HR_LRL + (deltaI_HR * 10 / React_Time));
      state Decrement_HR2
        deltaD_HR = floor((MSR + prev_HR_LRL)) / 2 - ReqD_HR_LRL;
        HR_LRLR = floor(prev_HR_LRL - (deltaD_HR * 10) / ( Recov_Time*60))
      state Maintain_HR2
        HR_LRLR = prev_HR_LRL;
      (default) -> VOOR.VOOR_CHARGE.Charge
      VOOR.VOOR_CHARGE.Charge -> ENTRY_STATE2
      ENTRY_STATE2 -> (junction 346) [order 1] : [Activ_Rate >= Act_Thresh]
      ENTRY_STATE2 -> (junction 345) [order 2] : [Activ_Rate< Act_Thresh]
      (junction 346) -> Maintain_HR2 [order 2] : [prev_HR_LRL >= ReqI_HR_LRL]
      (junction 346) -> Increment_HR2 [order 1] : [prev_HR_LRL < ReqI_HR_LRL]
      (junction 345) -> Maintain_HR2 [order 1] : [prev_HR_LRL <= ReqD_HR_LRL]
      (junction 345) -> Decrement_HR2 [order 2] : [prev_HR_LRL > ReqD_HR_LRL]
    state Pace
      entry:
      PACE_CHARGE_CTRL = false;
      PACE_GND_CTRL = true;
      ATR_PACE_CTRL = false;
      ATR_GND_CTRL = false;
      Z_ATR_CTRL = false;
      Z_VENT_CTRL = false;
      VENT_GND_CTRL = false;
      VENT_PACE_CTRL = true;
      %FRONTEND_CTRL = true;
    (default) -> VOOR_CHARGE : {HR_LRLR = HR_LRL}
    VOOR_CHARGE -> VOOR.Pace : [after((60000 / HR_LRLR - VPW), msec)]
    VOOR.Pace -> VOOR_CHARGE : [after(VPW, msec)]
  state AOOR
    state AOOR_Charge
      state CHARGE
        entry:
        ATR_PACE_CTRL = false;
        VENT_PACE_CTRL = false;
        PACING_REF_PWM = ATR_PWM_AMPLITUDE;
        PACE_CHARGE_CTRL = true;
        %Discharging Blocking Capacitor
        PACE_GND_CTRL = true;
        VENT_PACE_CTRL = false;
        Z_ATR_CTRL = false;
        Z_VENT_CTRL = false;
        %% ATR_PACE_CTRL = false;
        ATR_GND_CTRL = true;
        VENT_GND_CTRL = false;
        Activ_Rate = single(sqrt(abs(Activ(1))^2+abs(Activ(2))^2+abs(Activ(3))^2));
      state ENTRY_STATE1
        prev_HR_LRL = HR_LRLR;
        %% equation to get Reqi_HR_LRL
        ReqI_HR_LRL = ceil((MSR - HR_LRL) * (Resp_Fact / 16) + HR_LRL);
        %% Final_dHR is just HR_LRL
        ReqD_HR_LRL = HR_LRL;
      state Increment_HR1
        %% deltaI_HR = uint16(Activ_Rate * 10);
        deltaI_HR = ceil((ReqI_HR_LRL - prev_HR_LRL) + (uint16(round(Activ_Rate)) ));
        HR_LRLR = ceil(prev_HR_LRL + (deltaI_HR * 10 / React_Time));
      state Decrement_HR1
        deltaD_HR = floor((MSR + prev_HR_LRL)) / 2 - ReqD_HR_LRL;
        HR_LRLR = floor(prev_HR_LRL - (deltaD_HR * 10) / ( Recov_Time*60))
      state Maintain_HR1
        HR_LRLR = prev_HR_LRL;
      (default) -> AOOR.AOOR_Charge.CHARGE
      AOOR.AOOR_Charge.CHARGE -> AOOR.AOOR_Charge.ENTRY_STATE1
      AOOR.AOOR_Charge.ENTRY_STATE1 -> (junction 311) [order 1] : [Activ_Rate >= Act_Thresh]
      AOOR.AOOR_Charge.ENTRY_STATE1 -> (junction 322) [order 2] : [Activ_Rate< Act_Thresh]
      (junction 311) -> AOOR.AOOR_Charge.Maintain_HR1 [order 2] : [prev_HR_LRL >= ReqI_HR_LRL]
      (junction 311) -> AOOR.AOOR_Charge.Increment_HR1 [order 1] : [prev_HR_LRL < ReqI_HR_LRL]
      (junction 322) -> AOOR.AOOR_Charge.Maintain_HR1 [order 1] : [prev_HR_LRL <= ReqD_HR_LRL]
      (junction 322) -> AOOR.AOOR_Charge.Decrement_HR1 [order 2] : [prev_HR_LRL > ReqD_HR_LRL]
    state PACE
      entry:
      PACE_CHARGE_CTRL = false;
      PACE_GND_CTRL = true;
      ATR_PACE_CTRL = true;
      ATR_GND_CTRL = false;
      Z_ATR_CTRL = false;
      Z_VENT_CTRL = false;
      VENT_GND_CTRL = false;
      VENT_PACE_CTRL = false;
    (default) -> AOOR_Charge : {HR_LRLR = HR_LRL}
    AOOR_Charge -> PACE : [after((60000 / HR_LRLR - APW), msec)]
    PACE -> AOOR_Charge : [after(APW, msec)]
  Entry -> AOO [order 1] : [MODE == 1]
  AOO -> Entry : [MODE ~= 1]
  Entry -> VOO [order 2] : [MODE == 0]
  VOO -> Entry : [MODE ~= 0]
  (default) -> Entry
  Entry -> DOOR [order 10] : [MODE == 9]
  Entry -> AAI [order 4] : [MODE == 3]
  AAI -> Entry : [MODE ~= 3]
  DOOR -> Entry : [MODE ~= 9]
  Entry -> VVI [order 3] : [MODE == 2]
  Entry -> VVIR [order 9] : [MODE == 8]
  VVI -> Entry : [MODE ~= 2]
  VVIR -> Entry : [MODE ~= 8]
  Entry -> AAIR [order 7] : [MODE == 7]
  Entry -> DOO [order 5] : [MODE == 4]
  AAIR -> Entry : [MODE ~= 7]
  DOO -> Entry : [MODE ~= 4]
  VOOR -> Entry : [MODE ~= 5]
  Entry -> VOOR [order 8] : [MODE == 5]
  Entry -> AOOR [order 6] : [MODE == 6]
  AOOR -> Entry : [MODE ~= 6]
  data: MODE input uint8; FRONTEND_CTRL output boolean; delay local uint16; HR_LRL input uint16; URL input uint8; AVDelay input uint16; ATR_PWM_AMPLITUDE input uint8; VENT_PWM_AMPLITUDE input uint8; APW input uint16; VPW input uint16; VENT_CMP_REF_PWM output uint16; ATR_CMP_REF_PWM output uint16; ARP input uint16; VRP input uint16; PVARP input uint16; Rate_Smoothing input uint8; Act_Thresh input single; React_Time input uint16; Resp_Fact input uint16; Recov_Time input uint16; MSR input uint16; VENT_CMP_DETECT input boolean; ATR_CMP_DETECT input boolean; PACING_REF_PWM output uint8; ATR_PACE_CTRL output boolean; VENT_PACE_CTRL output boolean; PACE_CHARGE_CTRL output boolean; PACE_GND_CTRL output boolean; Z_ATR_CTRL output boolean; Z_VENT_CTRL output boolean; ATR_GND_CTRL output boolean; VENT_GND_CTRL output boolean; HR_LRLR local uint16; Activ input double; prev_HR_LRL local uint16; ReqI_HR_LRL local uint16; deltaI_HR local uint16; ReqD_HR_LRL local uint16; deltaD_HR local uint16; Activ_Rate local single
